simulink model "AppMain"  (R2023a)
settings: Solver=FixedStepDiscrete  StartTime=0.0  StopTime=0.02  FixedStep=10e-3  RelTol=1e-3
PreLoadFcn:
  | AppMain_data
values from neighbouring files (symbols this model uses):
  CtrlConst = struct    [AppMain_data.m]
  TaskTimeBase = struct    [AppMain_data.m]
libraries: simulink x23, lib1 x6
(part 2 of 2)

== system AppMain/FeedBack/Subsystem7/Subsystem5 ==
  FaultFlag : Inport  OutDataTypeStr=boolean
  FaultCnt : Inport  Port=2  OutDataTypeStr=uint8
  MotorRunEn : Inport  Port=3
  Compare To Constant : simulink/Logic and Bit Operations/Compare To Constant  relop=>=  const=2  OutDataTypeStr=boolean
  Logical Operator : Logic  AllPortsSameDT=off  OutDataTypeStr=boolean
  Logical Operator3 : Logic  AllPortsSameDT=off  OutDataTypeStr=boolean
  FeedBackEn : Outport  VectorParamsAs1DForOutWhenUnconnected=off
  wires:
  Compare To Constant/1 -> Logical Operator3/2
  Logical Operator3/1 -> Logical Operator/1
  Logical Operator/1 -> FeedBackEn/1
  MotorRunEn/1 -> Logical Operator/2
  FaultCnt/1 -> Compare To Constant/1
  FaultFlag/1 -> Logical Operator3/1

== system AppMain/FeedBack/Subsystem7/Subsystem6 ==
  FaultFlag : Inport  OutDataTypeStr=boolean
  MotorRunEn : Inport  Port=2
  MDryRunningCnt : Inport  Port=3  OutDataTypeStr=uint8
  Compare To Constant : simulink/Logic and Bit Operations/Compare To Constant  relop=>=  const=2  OutDataTypeStr=boolean
  Logical Operator : Logic  AllPortsSameDT=off  OutDataTypeStr=boolean
  Logical Operator3 : Logic  AllPortsSameDT=off  OutDataTypeStr=boolean
  FeedBackEn : Outport  VectorParamsAs1DForOutWhenUnconnected=off
  wires:
  MotorRunEn/1 -> Logical Operator/2
  Logical Operator/1 -> FeedBackEn/1
  FaultFlag/1 -> Logical Operator3/1
  Logical Operator3/1 -> Logical Operator/1
  Compare To Constant/1 -> Logical Operator3/2
  MDryRunningCnt/1 -> Compare To Constant/1

== system AppMain/MotorRestartAndFaultCnt/MotorFalutHandle/MotorFaultRecoverTimer ==
  RestartInterval : Inport  OutDataTypeStr=uint16
  MotorRestartCompleted : Inport  Port=2
  MotorRestartFSM : Stateflow chart  TreatAsAtomicUnit=on
  RecoverEnable : Outport  VectorParamsAs1DForOutWhenUnconnected=off
  wires:
  MotorRestartCompleted/1 -> MotorRestartFSM/2(MotorRestartCompleted)
  MotorRestartFSM/1(RecoverEn) -> RecoverEnable/1
  RestartInterval/1 -> MotorRestartFSM/1(TimeTHR)

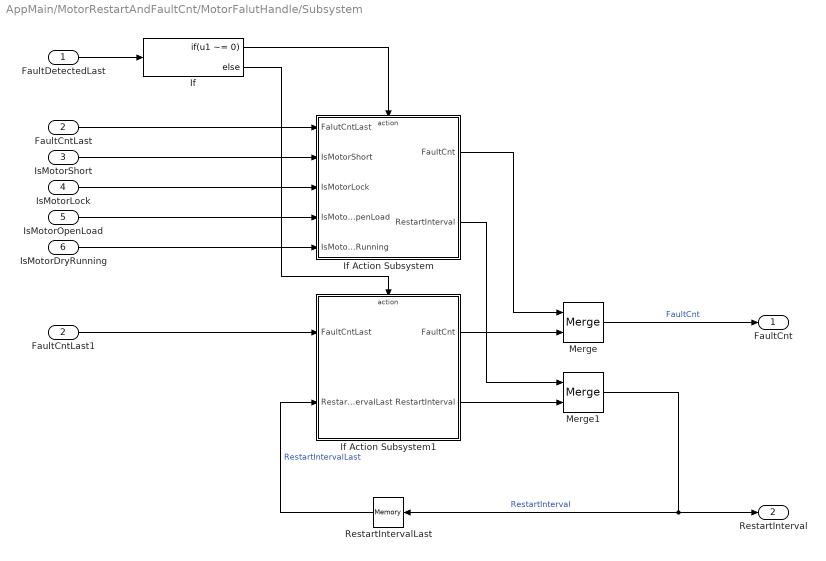
== system AppMain/MotorRestartAndFaultCnt/MotorFalutHandle/Subsystem ==
  FaultDetectedLast : Inport  OutDataTypeStr=boolean
  FaultCntLast : Inport  Port=2  OutDataTypeStr=Bus: MotorFaultCnt_t
  IsMotorShort : Inport  Port=3  OutDataTypeStr=boolean
  IsMotorLock : Inport  Port=4  OutDataTypeStr=boolean
  IsMotorOpenLoad : Inport  Port=5  OutDataTypeStr=boolean
  IsMotorDryRunning : Inport  Port=6  OutDataTypeStr=boolean
  FaultCntLast1 : InportShadow  Port=2  OutDataTypeStr=Bus: MotorFaultCnt_t
  If : If  IfExpression=u1 ~= 0
  If Action Subsystem : Subsystem  TreatAsAtomicUnit=on
  If Action Subsystem1 : Subsystem  TreatAsAtomicUnit=on
  Merge : Merge
  Merge1 : Merge
  RestartIntervalLast : Memory  InheritSampleTime=on
  FaultCnt : Outport  OutDataTypeStr=Bus: MotorFaultCnt_t  VectorParamsAs1DForOutWhenUnconnected=off
  RestartInterval : Outport  Port=2  OutDataTypeStr=uint16  VectorParamsAs1DForOutWhenUnconnected=off
  wires:
  RestartIntervalLast/1 -> If Action Subsystem1/2(RestartIntervalLast)  "RestartIntervalLast"
  If Action Subsystem1/2(RestartInterval) -> Merge1/2
  If Action Subsystem1/1(FaultCnt) -> Merge/2
  If/1 -> If Action Subsystem/Action
  If/2 -> If Action Subsystem1/Action
  Merge1/1 -> RestartIntervalLast/1, RestartInterval/1  "RestartInterval"
  FaultCntLast/1 -> If Action Subsystem/1(FalutCntLast)
  If Action Subsystem/1(FaultCnt) -> Merge/1
  Merge/1 -> FaultCnt/1  "FaultCnt"
  If Action Subsystem/2(RestartInterval) -> Merge1/1
  FaultDetectedLast/1 -> If/1
  IsMotorShort/1 -> If Action Subsystem/2(IsMotorShort)
  IsMotorLock/1 -> If Action Subsystem/3(IsMotorLock)
  IsMotorOpenLoad/1 -> If Action Subsystem/4(IsMotorOpenLoad)
  FaultCntLast1/1 -> If Action Subsystem1/1(FaultCntLast)
  IsMotorDryRunning/1 -> If Action Subsystem/5(IsMotorDryRunning)

== system AppMain/MotorRestartAndFaultCnt/MotorFalutHandle/Subsystem1 ==
  IsMotorShort : Inport  OutDataTypeStr=boolean
  IsMotorOpenLoad : Inport  Port=2  OutDataTypeStr=boolean
  TargetSpeed : Inport  Port=3  OutDataTypeStr=int16
  RestartEnable : Inport  Port=4  OutDataTypeStr=boolean
  IsMotorLock : Inport  Port=5  OutDataTypeStr=boolean
  If : If  NumInputs=2  IfExpression=u1 ~= 0  ElseIfExpressions=u2 ~= 0
  If Action Subsystem : Subsystem  TreatAsAtomicUnit=on
  If Action Subsystem1 : Subsystem  TreatAsAtomicUnit=on
  If Action Subsystem2 : Subsystem  TreatAsAtomicUnit=on
  Logical Operator : Logic  Operator=OR  AllPortsSameDT=off  OutDataTypeStr=boolean
  Merge : Merge  Inputs=3
  Scope : Scope
  Speed : Outport  OutDataTypeStr=int16  VectorParamsAs1DForOutWhenUnconnected=off
  wires:
  IsMotorShort/1 -> Logical Operator/1
  IsMotorOpenLoad/1 -> Logical Operator/2
  Logical Operator/1 -> If/1
  TargetSpeed/1 -> If Action Subsystem2/2(SpeedIn), If Action Subsystem1/1(SpeedIn), If Action Subsystem/1(SpeedIn)
  RestartEnable/1 -> If Action Subsystem2/1(RestartEnable), If Action Subsystem1/2(RestartEnable)
  If/1 -> If Action Subsystem/Action
  If Action Subsystem1/1(SpeedOut) -> Merge/2
  If Action Subsystem/1(SpeedOut) -> Merge/1
  Merge/1 -> Speed/1, Scope/1
  IsMotorLock/1 -> If/2
  If/2 -> If Action Subsystem1/Action
  If/3 -> If Action Subsystem2/Action
  If Action Subsystem2/1(SpeedOut) -> Merge/3

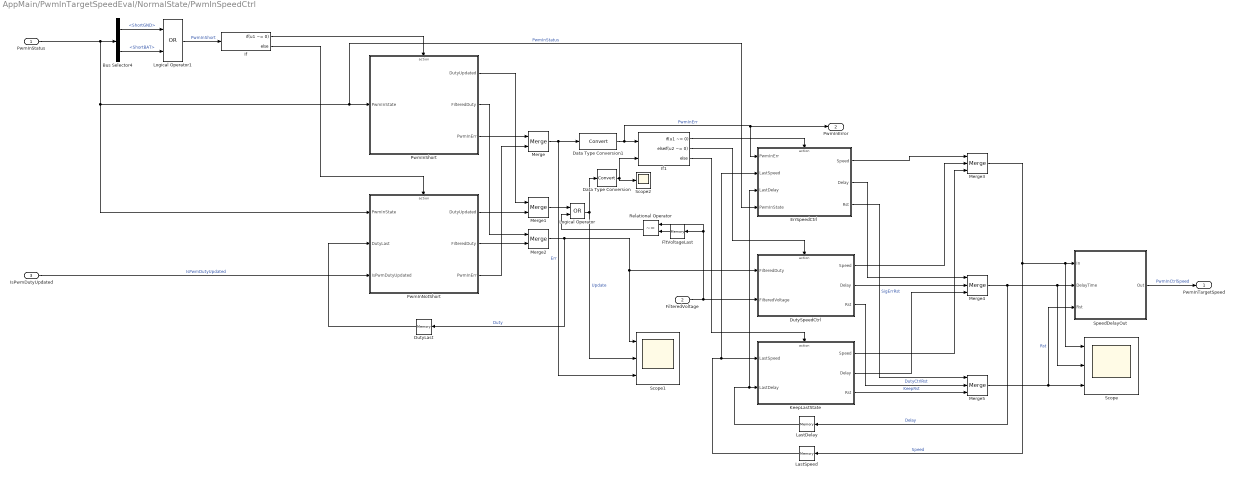
== system AppMain/PwmInTargetSpeedEval/NormalState/PwmInSpeedCtrl ==
  PwmInStatus : Inport
  FilteredVoltage : Inport  Port=2  OutDataTypeStr=int16
  IsPwmDutyUpdated : Inport  Port=3  OutDataTypeStr=boolean
  Bus Selector4 : BusSelector  OutputSignals=ShortGND,ShortBAT
  Data Type Conversion : DataTypeConversion  SaturateOnIntegerOverflow=off  RndMeth=Floor
  Data Type Conversion1 : DataTypeConversion  SaturateOnIntegerOverflow=off  RndMeth=Floor
  DutyLast : Memory  InitialCondition=CtrlConst.SpeedCtrl.PwmIn.Duty.Default  InheritSampleTime=on
  DutySpeedCtrl : Subsystem  TreatAsAtomicUnit=on
  ErrSpeedCtrl : Subsystem  TreatAsAtomicUnit=on
  FltVoltageLast : Memory  InheritSampleTime=on
  If : If  IfExpression=u1 ~= 0
  If1 : If  NumInputs=2  IfExpression=u1 ~= 0  ElseIfExpressions=u2 ~= 0
  KeepLastState : Subsystem  TreatAsAtomicUnit=on
  LastDelay : Memory  InheritSampleTime=on
  LastSpeed : Memory  InheritSampleTime=on
  Logical Operator : Logic  Operator=OR  AllPortsSameDT=off  OutDataTypeStr=boolean
  Logical Operator1 : Logic  Operator=OR  AllPortsSameDT=off  OutDataTypeStr=boolean
  Merge : Merge
  Merge1 : Merge
  Merge2 : Merge
  Merge3 : Merge  Inputs=3
  Merge4 : Merge  Inputs=3
  Merge5 : Merge  Inputs=3
  PwmInNotShort : Subsystem  TreatAsAtomicUnit=on
      settings: RTWSystemCode=Nonreusable function  RTWFcnNameOpts=Use subsystem name  FunctionInterfaceSpec=Allow arguments (Optimized)
  PwmInShort : Subsystem  TreatAsAtomicUnit=on
      settings: RTWSystemCode=Nonreusable function  RTWFcnNameOpts=Use subsystem name  FunctionInterfaceSpec=Allow arguments (Optimized)
  Relational Operator : RelationalOperator  Operator=~=  OutDataTypeStr=boolean  RndMeth=Simplest  InputSameDT=off
  Scope : Scope  NumInputPorts=3
  Scope1 : Scope  NumInputPorts=3
  Scope2 : Scope
  SpeedDelayOut : Subsystem  TreatAsAtomicUnit=on
      settings: RTWFcnNameOpts=Use subsystem name
  PwmInTargetSpeed : Outport  VectorParamsAs1DForOutWhenUnconnected=off
  PwmInError : Outport  Port=2  OutDataTypeStr=boolean  VectorParamsAs1DForOutWhenUnconnected=off
  wires:
  SpeedDelayOut/1(Out) -> PwmInTargetSpeed/1  "PwmInCtrlSpeed"
  PwmInStatus/1 -> PwmInNotShort/1(PwmInState), ErrSpeedCtrl/4(PwmInState), PwmInShort/1(PwmInState), Bus Selector4/1  "PwmInStatus"
  Bus Selector4/1 -> Logical Operator1/1  "<ShortGND>"
  Bus Selector4/2 -> Logical Operator1/2  "<ShortBAT>"
  Logical Operator1/1 -> If/1  "PwmInShort"
  If/1 -> PwmInShort/Action
  If/2 -> PwmInNotShort/Action
  PwmInShort/3(PwmInErr) -> Merge/1
  PwmInNotShort/3(PwmInErr) -> Merge/2
  If1/1 -> ErrSpeedCtrl/Action
  PwmInNotShort/1(DutyUpdated) -> Merge1/2
  PwmInShort/1(DutyUpdated) -> Merge1/1
  PwmInNotShort/2(FilteredDuty) -> Merge2/2
  PwmInShort/2(FilteredDuty) -> Merge2/1
  Merge2/1 -> DutyLast/1, Scope1/1, DutySpeedCtrl/1(FilteredDuty)  "Duty"
  ErrSpeedCtrl/1(Speed) -> Merge3/1
  DutySpeedCtrl/1(Speed) -> Merge3/2
  ErrSpeedCtrl/2(Delay) -> Merge4/1
  DutySpeedCtrl/2(Delay) -> Merge4/2
  ErrSpeedCtrl/3(Rst) -> Merge5/1  "SigErrRst"
  DutySpeedCtrl/3(Rst) -> Merge5/2  "DutyCtrlRst"
  Merge3/1 -> SpeedDelayOut/1(In), Scope/1, LastSpeed/1  "Speed"
  Merge4/1 -> Scope/2, SpeedDelayOut/2(DelayTime), LastDelay/1  "Delay"
  Merge5/1 -> Scope/3, SpeedDelayOut/3(Rst)  "Rst"
  If1/2 -> DutySpeedCtrl/Action
  Merge1/1 -> Logical Operator/1
  If1/3 -> KeepLastState/Action
  LastDelay/1 -> ErrSpeedCtrl/3(LastDelay), KeepLastState/2(LastDelay)
  LastSpeed/1 -> ErrSpeedCtrl/2(LastSpeed), KeepLastState/1(LastSpeed)
  KeepLastState/3(Rst) -> Merge5/3  "KeepRst"
  KeepLastState/2(Delay) -> Merge4/3
  KeepLastState/1(Speed) -> Merge3/3
  Data Type Conversion1/1 -> ErrSpeedCtrl/1(PwmInErr), PwmInError/1, If1/1  "PwmInErr"
  Data Type Conversion/1 -> If1/2, Scope2/1
  DutyLast/1 -> PwmInNotShort/2(DutyLast)
  FltVoltageLast/1 -> Relational Operator/2
  FilteredVoltage/1 -> FltVoltageLast/1, Relational Operator/1, DutySpeedCtrl/2(FilteredVoltage)
  Relational Operator/1 -> Logical Operator/2
  Merge/1 -> Data Type Conversion1/1, Scope1/3  "Err"
  Logical Operator/1 -> Scope1/2, Data Type Conversion/1  "Update"
  IsPwmDutyUpdated/1 -> PwmInNotShort/3(IsPwmDutyUpdated)  "IsPwmDutyUpdated"

== system AppMain/MotorRestartAndFaultCnt/MotorFalutHandle/Subsystem/If Action Subsystem ==
  FalutCntLast : Inport  OutDataTypeStr=Bus: MotorFaultCnt_t
  IsMotorShort : Inport  Port=2  OutDataTypeStr=boolean
  IsMotorLock : Inport  Port=3  OutDataTypeStr=boolean
  IsMotorOpenLoad : Inport  Port=4  OutDataTypeStr=boolean
  IsMotorDryRunning : Inport  Port=5  OutDataTypeStr=boolean
  Action Port : ActionPort  InitializeStates=reset  ActionPortLabel=if(u1 ~= 0)
  FaultCntIncrement : Subsystem
  RestartIntervalCaculate : Subsystem
  FaultCnt : Outport  OutDataTypeStr=Bus: MotorFaultCnt_t  VectorParamsAs1DForOutWhenUnconnected=off
  RestartInterval : Outport  Port=2  OutDataTypeStr=uint16  VectorParamsAs1DForOutWhenUnconnected=off
  wires:
  FaultCntIncrement/1(FaultCnt) -> RestartIntervalCaculate/1(MotorFaultCnt), FaultCnt/1
  FalutCntLast/1 -> FaultCntIncrement/1(FalutCntLast)
  IsMotorShort/1 -> FaultCntIncrement/2(IsMotorShort)
  RestartIntervalCaculate/1(TimeTHR) -> RestartInterval/1
  IsMotorOpenLoad/1 -> FaultCntIncrement/3(IsMotorOpenLoad)
  IsMotorLock/1 -> FaultCntIncrement/4(IsMotorLock)
  IsMotorDryRunning/1 -> FaultCntIncrement/5(IsMotorDryRunning)

== system AppMain/MotorRestartAndFaultCnt/MotorFalutHandle/Subsystem/If Action Subsystem1 ==
  FaultCntLast : Inport  OutDataTypeStr=Bus: MotorFaultCnt_t
  RestartIntervalLast : Inport  Port=2  OutDataTypeStr=uint16
  Action Port : ActionPort  InitializeStates=reset  ActionPortLabel=else
  Bus Creator : BusCreator  Inputs=4  OutDataTypeStr=Bus: MotorFaultCnt_t  NonVirtualBus=on
      settings: InheritFromInputs=off
  Bus Selector : BusSelector  OutputSignals=Short,Open,Lock,DryRunning
  FaultCnt : Outport  OutDataTypeStr=Bus: MotorFaultCnt_t  VectorParamsAs1DForOutWhenUnconnected=off
  RestartInterval : Outport  Port=2  OutDataTypeStr=uint16  VectorParamsAs1DForOutWhenUnconnected=off
  wires:
  FaultCntLast/1 -> Bus Selector/1
  Bus Creator/1 -> FaultCnt/1
  Bus Selector/1 -> Bus Creator/1  "<Short>"
  Bus Selector/2 -> Bus Creator/2  "<Open>"
  Bus Selector/3 -> Bus Creator/3  "<Lock>"
  RestartIntervalLast/1 -> RestartInterval/1
  Bus Selector/4 -> Bus Creator/4  "<DryRunning>"

== system AppMain/MotorRestartAndFaultCnt/MotorFalutHandle/Subsystem1/If Action Subsystem ==
  SpeedIn : Inport
  Action Port : ActionPort  ActionPortLabel=if(u1 ~= 0)
  SpeedOut : Outport  VectorParamsAs1DForOutWhenUnconnected=off
  wires:
  SpeedIn/1 -> SpeedOut/1

== system AppMain/MotorRestartAndFaultCnt/MotorFalutHandle/Subsystem1/If Action Subsystem1 ==
  SpeedIn : Inport
  RestartEnable : Inport  Port=2  OutDataTypeStr=boolean
  Action Port : ActionPort  InitializeStates=reset  ActionPortLabel=elseif(u2 ~= 0)
  Add : Sum  SaturateOnIntegerOverflow=on
  Compare To Constant : simulink/Logic and Bit Operations/Compare To Constant  relop=<=  const=2/5e-3  OutDataTypeStr=boolean
  Constant : Constant  Value=0  OutDataTypeStr=uint16
  Constant1 : Constant  OutDataTypeStr=uint16
  Constant2 : Constant  Value=-1000  OutDataTypeStr=int16
  Detect Increase : simulink/Logic and Bit Operations/Detect Increase  vinit=0.0  OutDataTypeStr=boolean
  Memory : Memory  InitialCondition=uint16(0)  InheritSampleTime=on
  Scope : Scope  NumInputPorts=2
  Switch : Switch  Criteria=u2 > Threshold  SaturateOnIntegerOverflow=off  InputSameDT=off
  Switch1 : Switch  Criteria=u2 > Threshold  SaturateOnIntegerOverflow=off  InputSameDT=off
  SpeedOut : Outport  VectorParamsAs1DForOutWhenUnconnected=off
  wires:
  RestartEnable/1 -> Detect Increase/1
  Detect Increase/1 -> Switch/2
  Switch/1 -> Memory/1, Compare To Constant/1
  Memory/1 -> Add/2
  Constant/1 -> Switch/1
  Add/1 -> Switch/3
  Constant1/1 -> Add/1
  Compare To Constant/1 -> Switch1/2, Scope/2
  Constant2/1 -> Switch1/1
  Switch1/1 -> SpeedOut/1, Scope/1
  SpeedIn/1 -> Switch1/3

== system AppMain/MotorRestartAndFaultCnt/MotorFalutHandle/Subsystem1/If Action Subsystem2 ==
  RestartEnable : Inport  OutDataTypeStr=boolean
  SpeedIn : Inport  Port=2
  Action Port : ActionPort  InitializeStates=reset  ActionPortLabel=else
  Constant : Constant  Value=0  OutDataTypeStr=int16
  Switch : Switch  Criteria=u2 > Threshold  SaturateOnIntegerOverflow=off  InputSameDT=off
  SpeedOut : Outport  VectorParamsAs1DForOutWhenUnconnected=off
  wires:
  Switch/1 -> SpeedOut/1
  Constant/1 -> Switch/3
  RestartEnable/1 -> Switch/2
  SpeedIn/1 -> Switch/1

== system AppMain/PwmInTargetSpeedEval/NormalState/PwmInSpeedCtrl/DutySpeedCtrl ==
  FilteredDuty : Inport  OutDataTypeStr=uint16
  FilteredVoltage : Inport  Port=2  OutDataTypeStr=int16
  Action Port : ActionPort  InitializeStates=reset  ActionPortLabel=elseif(u2 ~= 0)
  Scope : Scope
  SpeedAndOutDelayEval : Subsystem
      settings: RTWFcnNameOpts=Use subsystem name
  Speed : Outport  OutDataTypeStr=int16  VectorParamsAs1DForOutWhenUnconnected=off
  Delay : Outport  Port=2  OutDataTypeStr=uint16  VectorParamsAs1DForOutWhenUnconnected=off
  Rst : Outport  Port=3  OutDataTypeStr=boolean  VectorParamsAs1DForOutWhenUnconnected=off
  wires:
  FilteredDuty/1 -> SpeedAndOutDelayEval/1(FilteredDuty)
  SpeedAndOutDelayEval/1(DutySpeed) -> Speed/1  "Speed"
  SpeedAndOutDelayEval/2(DelayTime) -> Delay/1  "Delay"
  SpeedAndOutDelayEval/3(DelayRst) -> Rst/1, Scope/1  "Rst"
  FilteredVoltage/1 -> SpeedAndOutDelayEval/2(FilteredVoltage)

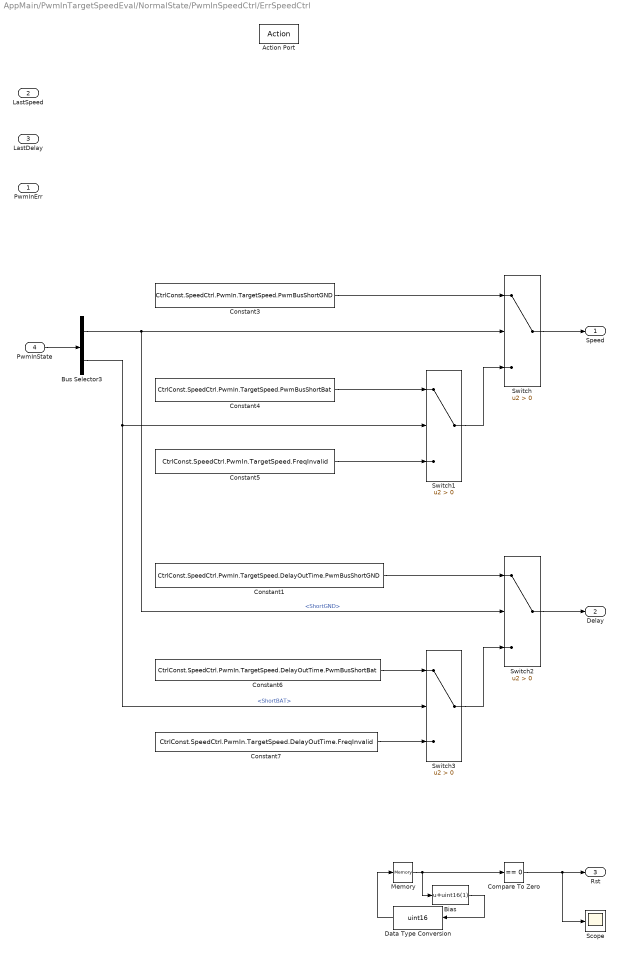
== system AppMain/PwmInTargetSpeedEval/NormalState/PwmInSpeedCtrl/ErrSpeedCtrl ==
  PwmInErr : Inport  OutDataTypeStr=boolean
  LastSpeed : Inport  Port=2  OutDataTypeStr=int16
  LastDelay : Inport  Port=3  OutDataTypeStr=uint16
  PwmInState : Inport  Port=4
  Action Port : ActionPort  InitializeStates=reset  ActionPortLabel=if(u1 ~= 0)
  Bias : Bias  Bias=uint16(1)  SaturateOnIntegerOverflow=off
  Bus Selector3 : BusSelector  OutputSignals=ShortGND,ShortBAT
  Compare To Zero : simulink/Logic and Bit Operations/Compare To Zero  relop===  OutDataTypeStr=boolean
  Constant1 : Constant  Value=CtrlConst.SpeedCtrl.PwmIn.TargetSpeed.DelayOutTime.PwmBusShortGND
  Constant3 : Constant  Value=CtrlConst.SpeedCtrl.PwmIn.TargetSpeed.PwmBusShortGND
  Constant4 : Constant  Value=CtrlConst.SpeedCtrl.PwmIn.TargetSpeed.PwmBusShortBat
  Constant5 : Constant  Value=CtrlConst.SpeedCtrl.PwmIn.TargetSpeed.FreqInvalid
  Constant6 : Constant  Value=CtrlConst.SpeedCtrl.PwmIn.TargetSpeed.DelayOutTime.PwmBusShortBat
  Constant7 : Constant  Value=CtrlConst.SpeedCtrl.PwmIn.TargetSpeed.DelayOutTime.FreqInvalid
  Data Type Conversion : DataTypeConversion  OutDataTypeStr=uint16  SaturateOnIntegerOverflow=off  RndMeth=Floor
  Memory : Memory  InitialCondition=uint16(0)  InheritSampleTime=on
  Scope : Scope
  Switch{,1..3} (4 alike) : Switch  Criteria=u2 > Threshold  SaturateOnIntegerOverflow=off  InputSameDT=off
  Speed : Outport  OutDataTypeStr=int16  VectorParamsAs1DForOutWhenUnconnected=off
  Delay : Outport  Port=2  OutDataTypeStr=uint16  VectorParamsAs1DForOutWhenUnconnected=off
  Rst : Outport  Port=3  OutDataTypeStr=boolean  VectorParamsAs1DForOutWhenUnconnected=off
  wires:
  PwmInState/1 -> Bus Selector3/1
  Constant3/1 -> Switch/1
  Switch1/1 -> Switch/3
  Constant4/1 -> Switch1/1
  Constant5/1 -> Switch1/3
  Switch/1 -> Speed/1
  Switch3/1 -> Switch2/3
  Bus Selector3/2 -> Switch3/2, Switch1/2  "<ShortBAT>"
  Constant1/1 -> Switch2/1
  Bus Selector3/1 -> Switch2/2, Switch/2  "<ShortGND>"
  Constant7/1 -> Switch3/3
  Constant6/1 -> Switch3/1
  Switch2/1 -> Delay/1
  Data Type Conversion/1 -> Memory/1
  Bias/1 -> Data Type Conversion/1
  Memory/1 -> Bias/1, Compare To Zero/1
  Compare To Zero/1 -> Rst/1, Scope/1

== system AppMain/PwmInTargetSpeedEval/NormalState/PwmInSpeedCtrl/KeepLastState ==
  LastSpeed : Inport  OutDataTypeStr=int16
  LastDelay : Inport  Port=2  OutDataTypeStr=uint16
  Action Port : ActionPort  InitializeStates=reset  ActionPortLabel=else
  Constant : Constant  Value=false  OutDataTypeStr=boolean
  Speed : Outport  OutDataTypeStr=int16  VectorParamsAs1DForOutWhenUnconnected=off
  Delay : Outport  Port=2  OutDataTypeStr=uint16  VectorParamsAs1DForOutWhenUnconnected=off
  Rst : Outport  Port=3  OutDataTypeStr=boolean  VectorParamsAs1DForOutWhenUnconnected=off
  wires:
  LastSpeed/1 -> Speed/1
  LastDelay/1 -> Delay/1
  Constant/1 -> Rst/1

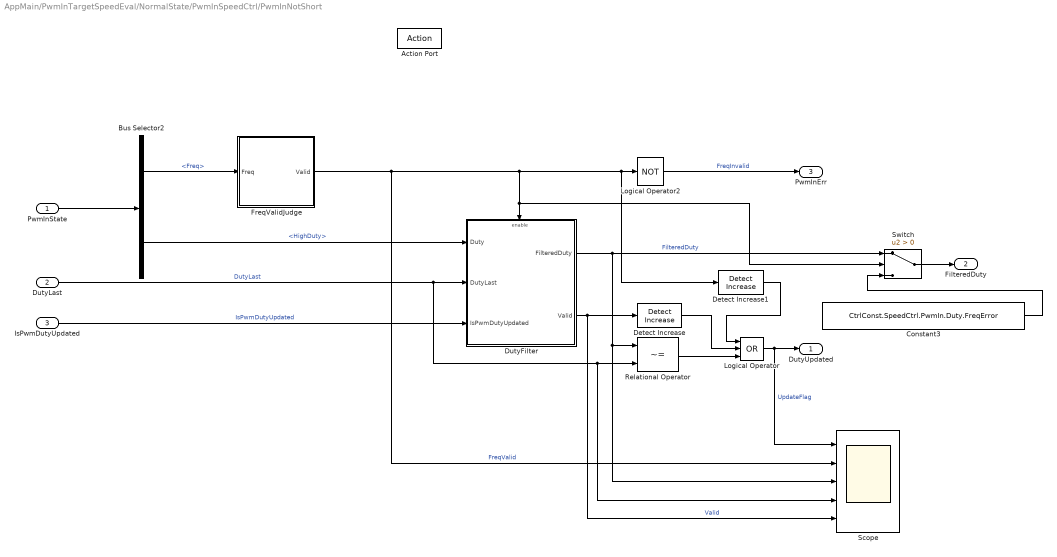
== system AppMain/PwmInTargetSpeedEval/NormalState/PwmInSpeedCtrl/PwmInNotShort ==
  PwmInState : Inport
  DutyLast : Inport  Port=2  OutDataTypeStr=uint16
  IsPwmDutyUpdated : Inport  Port=3  OutDataTypeStr=boolean
  Action Port : ActionPort  InitializeStates=reset  ActionPortLabel=else
  Bus Selector2 : BusSelector  OutputSignals=Freq,HighDuty
  Constant3 : Constant  Value=CtrlConst.SpeedCtrl.PwmIn.Duty.FreqError
  Detect Increase : simulink/Logic and Bit Operations/Detect Increase  vinit=0.0  OutDataTypeStr=boolean
  Detect Increase1 : simulink/Logic and Bit Operations/Detect Increase  vinit=0.0  OutDataTypeStr=boolean
  DutyFilter : Subsystem  TreatAsAtomicUnit=on
      settings: RTWFcnNameOpts=Use subsystem name
  FreqValidJudge : Subsystem  TreatAsAtomicUnit=on
      settings: RTWFcnNameOpts=Use subsystem name
  Logical Operator : Logic  Operator=OR  Inputs=3  AllPortsSameDT=off  OutDataTypeStr=boolean
  Logical Operator2 : Logic  Operator=NOT  Inputs=3  AllPortsSameDT=off  OutDataTypeStr=boolean
  Relational Operator : RelationalOperator  Operator=~=  OutDataTypeStr=boolean  RndMeth=Simplest  InputSameDT=off
  Scope : Scope  NumInputPorts=5
  Switch : Switch  Criteria=u2 > Threshold  SaturateOnIntegerOverflow=off  InputSameDT=off
  DutyUpdated : Outport  OutDataTypeStr=boolean  VectorParamsAs1DForOutWhenUnconnected=off
  FilteredDuty : Outport  Port=2  OutDataTypeStr=uint16  VectorParamsAs1DForOutWhenUnconnected=off
  PwmInErr : Outport  Port=3  OutDataTypeStr=boolean  VectorParamsAs1DForOutWhenUnconnected=off
  wires:
  Detect Increase/1 -> Logical Operator/2
  DutyFilter/2(Valid) -> Scope/5, Detect Increase/1  "Valid"
  PwmInState/1 -> Bus Selector2/1
  Bus Selector2/2 -> DutyFilter/1(Duty)  "<HighDuty>"
  Bus Selector2/1 -> FreqValidJudge/1(Freq)  "<Freq>"
  DutyFilter/1(FilteredDuty) -> Switch/1, Relational Operator/1, Scope/3  "FilteredDuty"
  Logical Operator2/1 -> PwmInErr/1  "FreqInvalid"
  FreqValidJudge/1(Valid) -> Detect Increase1/1, Logical Operator2/1, Switch/2, DutyFilter/Enable, Scope/2  "FreqValid"
  DutyLast/1 -> Relational Operator/2, Scope/4, DutyFilter/2(DutyLast)  "DutyLast"
  Relational Operator/1 -> Logical Operator/3
  Logical Operator/1 -> DutyUpdated/1, Scope/1  "UpdateFlag"
  IsPwmDutyUpdated/1 -> DutyFilter/3(IsPwmDutyUpdated)  "IsPwmDutyUpdated"
  Detect Increase1/1 -> Logical Operator/1
  Switch/1 -> FilteredDuty/1
  Constant3/1 -> Switch/3

== system AppMain/PwmInTargetSpeedEval/NormalState/PwmInSpeedCtrl/PwmInShort ==
  PwmInState : Inport
  Action Port : ActionPort  InitializeStates=reset  ActionPortLabel=if(u1 ~= 0)
  Bus Selector3 : BusSelector  OutputSignals=ShortGND,ShortBAT
  Constant : Constant  OutDataTypeStr=boolean
  Detect Increase : simulink/Logic and Bit Operations/Detect Increase  vinit=0.0  OutDataTypeStr=boolean
  Detect Increase1 : simulink/Logic and Bit Operations/Detect Increase  vinit=0.0  OutDataTypeStr=boolean
  Duty0 : Constant  Value=0  OutDataTypeStr=uint16
  Duty100 : Constant  Value=1000  OutDataTypeStr=uint16
  Logical Operator3 : Logic  Operator=OR  AllPortsSameDT=off  OutDataTypeStr=boolean
  Switch : Switch  Criteria=u2 > Threshold  SaturateOnIntegerOverflow=off  InputSameDT=off
  DutyUpdated : Outport  OutDataTypeStr=boolean  VectorParamsAs1DForOutWhenUnconnected=off
  FilteredDuty : Outport  Port=2  OutDataTypeStr=uint16  VectorParamsAs1DForOutWhenUnconnected=off
  PwmInErr : Outport  Port=3  OutDataTypeStr=boolean  VectorParamsAs1DForOutWhenUnconnected=off
  wires:
  Switch/1 -> FilteredDuty/1  "FilteredDuty"
  Logical Operator3/1 -> DutyUpdated/1  "DutyUpdate"
  Bus Selector3/2 -> Detect Increase1/1, Switch/2  "<ShortBAT>"
  Bus Selector3/1 -> Detect Increase/1  "<ShortGND>"
  Detect Increase1/1 -> Logical Operator3/2
  Detect Increase/1 -> Logical Operator3/1
  Duty0/1 -> Switch/3
  Duty100/1 -> Switch/1
  PwmInState/1 -> Bus Selector3/1
  Constant/1 -> PwmInErr/1

== system AppMain/PwmInTargetSpeedEval/NormalState/PwmInSpeedCtrl/SpeedDelayOut ==
  In : Inport
  DelayTime : Inport  Port=2
  Rst : Inport  Port=3
  DelayOut : Stateflow chart  TreatAsAtomicUnit=on
  OutLast : Memory  InheritSampleTime=on
  Out : Outport  VectorParamsAs1DForOutWhenUnconnected=off
  wires:
  In/1 -> DelayOut/1(In)  "In"
  OutLast/1 -> DelayOut/4(OutLast)  "OutLast"
  Rst/1 -> DelayOut/3(Rst)  "Rst"
  DelayOut/1(Out) -> OutLast/1, Out/1  "Out"
  DelayTime/1 -> DelayOut/2(DelayTHR)  "DelayTHR"

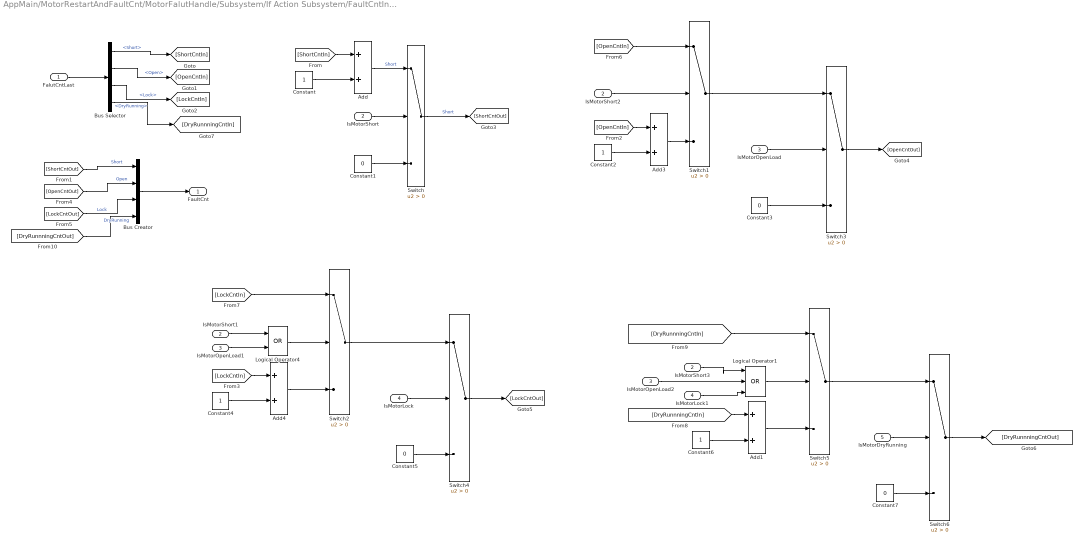
== system AppMain/MotorRestartAndFaultCnt/MotorFalutHandle/Subsystem/If Action Subsystem/FaultCntIncrement ==
  FalutCntLast : Inport  OutDataTypeStr=Bus: MotorFaultCnt_t
  IsMotorShort : Inport  Port=2  OutDataTypeStr=boolean
  IsMotorOpenLoad : Inport  Port=3  OutDataTypeStr=boolean
  IsMotorLock : Inport  Port=4  OutDataTypeStr=boolean
  IsMotorDryRunning : Inport  Port=5  OutDataTypeStr=boolean
  Add{,1,3..4} (4 alike) : Sum  SaturateOnIntegerOverflow=on
  Bus Creator : BusCreator  Inputs=4  OutDataTypeStr=Bus: MotorFaultCnt_t  NonVirtualBus=on
      settings: InheritFromInputs=off
  Bus Selector : BusSelector  OutputSignals=Short,Open,Lock,DryRunning
  Constant{,2,4,6} (4 alike) : Constant  OutDataTypeStr=uint8
  Constant{1,3,5,7} (4 alike) : Constant  Value=0  OutDataTypeStr=uint8
  IsMotorLock1 : InportShadow  Port=4  OutDataTypeStr=boolean
  IsMotorOpenLoad1 : InportShadow  Port=3  OutDataTypeStr=boolean
  IsMotorOpenLoad2 : InportShadow  Port=3  OutDataTypeStr=boolean
  IsMotorShort1 : InportShadow  Port=2  OutDataTypeStr=boolean
  IsMotorShort2 : InportShadow  Port=2  OutDataTypeStr=boolean
  IsMotorShort3 : InportShadow  Port=2  OutDataTypeStr=boolean
  Logical Operator1 : Logic  Operator=OR  Inputs=3  AllPortsSameDT=off  OutDataTypeStr=boolean
  Logical Operator4 : Logic  Operator=OR  AllPortsSameDT=off  OutDataTypeStr=boolean
  Switch{,1..6} (7 alike) : Switch  Criteria=u2 > Threshold  SaturateOnIntegerOverflow=off  InputSameDT=off
  FaultCnt : Outport  OutDataTypeStr=Bus: MotorFaultCnt_t  VectorParamsAs1DForOutWhenUnconnected=off
  wires:
  Bus Creator/1 -> FaultCnt/1
  Constant/1 -> Add/2
  Bus Selector/2 -> [OpenCntIn]  "<Open>"
  Bus Selector/1 -> [ShortCntIn]  "<Short>"
  Constant1/1 -> Switch/3
  Add/1 -> Switch/1  "Short"
  FalutCntLast/1 -> Bus Selector/1
  IsMotorShort/1 -> Switch/2
  Bus Selector/3 -> [LockCntIn]  "<Lock>"
  [ShortCntIn] -> Add/1
  Switch/1 -> [ShortCntOut]  "Short"
  [ShortCntOut] -> Bus Creator/1  "Short"
  Add3/1 -> Switch1/3
  Constant2/1 -> Add3/2
  [OpenCntIn] -> Add3/1
  Constant3/1 -> Switch3/3
  Switch3/1 -> [OpenCntOut]
  IsMotorShort1/1 -> Logical Operator4/1
  Switch4/1 -> [LockCntOut]
  [LockCntIn] -> Add4/1
  Constant4/1 -> Add4/2
  Constant5/1 -> Switch4/3
  IsMotorOpenLoad1/1 -> Logical Operator4/2
  [OpenCntOut] -> Bus Creator/2  "Open"
  [LockCntOut] -> Bus Creator/3  "Lock"
  IsMotorOpenLoad/1 -> Switch3/2
  IsMotorShort2/1 -> Switch1/2
  [OpenCntIn] -> Switch1/1
  Switch1/1 -> Switch3/1
  IsMotorLock/1 -> Switch4/2
  Switch2/1 -> Switch4/1
  Logical Operator4/1 -> Switch2/2
  [LockCntIn] -> Switch2/1
  Add4/1 -> Switch2/3
  Add1/1 -> Switch5/3
  Logical Operator1/1 -> Switch5/2
  [DryRunnningCntIn] -> Switch5/1
  [DryRunnningCntIn] -> Add1/1
  IsMotorDryRunning/1 -> Switch6/2
  Constant7/1 -> Switch6/3
  Switch5/1 -> Switch6/1
  Constant6/1 -> Add1/2
  Switch6/1 -> [DryRunnningCntOut]
  IsMotorShort3/1 -> Logical Operator1/1
  IsMotorLock1/1 -> Logical Operator1/3
  IsMotorOpenLoad2/1 -> Logical Operator1/2
  Bus Selector/4 -> [DryRunnningCntIn]  "<DryRunning>"
  [DryRunnningCntOut] -> Bus Creator/4  "DryRunning"

== system AppMain/MotorRestartAndFaultCnt/MotorFalutHandle/Subsystem/If Action Subsystem/RestartIntervalCaculate ==
  MotorFaultCnt : Inport  OutDataTypeStr=Bus: MotorFaultCnt_t
  Bus Selector : BusSelector  OutputSignals=Short,Open,Lock,DryRunning
  Dryrunning : Subsystem  TreatAsAtomicUnit=on
  If : If  NumInputs=3  ElseIfExpressions=u2 > 0,u3 > 0
  Lock : Subsystem  TreatAsAtomicUnit=on
  Merge : Merge  Inputs=4
  Open : Subsystem  TreatAsAtomicUnit=on
  Scope : Scope  NumInputPorts=4
  Short : Subsystem  TreatAsAtomicUnit=on
  TimeTHR : Outport  OutDataTypeStr=uint16  VectorParamsAs1DForOutWhenUnconnected=off
  wires:
  Bus Selector/1 -> If/1, Scope/2, Short/1(FaultCnt)  "<Short>"
  Bus Selector/3 -> Lock/1(FaultCnt), Scope/4, If/3  "<Lock>"
  Bus Selector/2 -> Open/1(FaultCnt), Scope/3, If/2  "<Open>"
  MotorFaultCnt/1 -> Bus Selector/1
  If/1 -> Short/Action
  If/2 -> Open/Action
  Merge/1 -> TimeTHR/1, Scope/1
  Open/1(Interval) -> Merge/2
  Lock/1(Interval) -> Merge/3
  Short/1(Interval) -> Merge/1
  If/3 -> Lock/Action
  If/4 -> Dryrunning/Action
  Bus Selector/4 -> Dryrunning/1(FaultCnt)  "<DryRunning>"
  Dryrunning/1(Interval) -> Merge/4

== system AppMain/PwmInTargetSpeedEval/NormalState/PwmInSpeedCtrl/DutySpeedCtrl/SpeedAndOutDelayEval ==
  FilteredDuty : Inport
  FilteredVoltage : Inport  Port=2  OutDataTypeStr=int16
  Constant : Constant  Value=CtrlConst.SpeedCtrl.PwmIn.TargetSpeed.Min  OutDataTypeStr=int16
  Data Type Conversion : DataTypeConversion  OutDataTypeStr=uint16  SaturateOnIntegerOverflow=off  RndMeth=Floor
  LastState : Memory  InitialCondition=uint16(0)  InheritSampleTime=on
  MaxSpeedLimtedByVoltage : Subsystem  TreatAsAtomicUnit=on
  SpeedCurve : MATLAB Function  TreatAsAtomicUnit=on
      settings: RTWFcnNameOpts=Use subsystem name
  DutySpeed : Outport  VectorParamsAs1DForOutWhenUnconnected=off
  DelayTime : Outport  Port=2  VectorParamsAs1DForOutWhenUnconnected=off
  DelayRst : Outport  Port=3  OutDataTypeStr=boolean  VectorParamsAs1DForOutWhenUnconnected=off
  wires:
  FilteredDuty/1 -> SpeedCurve/3(Duty)  "FilteredDuty"
  LastState/1 -> Data Type Conversion/1
  SpeedCurve/4(SectorNew) -> LastState/1
  SpeedCurve/1(Speed) -> DutySpeed/1
  SpeedCurve/2(Delay) -> DelayTime/1
  SpeedCurve/3(Reset) -> DelayRst/1
  Data Type Conversion/1 -> SpeedCurve/4(SectorLast)
  MaxSpeedLimtedByVoltage/1(MaxSpeed) -> SpeedCurve/1(MaxSpeed)
  FilteredVoltage/1 -> MaxSpeedLimtedByVoltage/1(Voltage)
  Constant/1 -> SpeedCurve/2(MinSpeed)

== system AppMain/PwmInTargetSpeedEval/NormalState/PwmInSpeedCtrl/PwmInNotShort/DutyFilter ==
  Duty : Inport
  DutyLast : Inport  Port=2  OutDataTypeStr=uint16
  IsPwmDutyUpdated : Inport  Port=3  OutDataTypeStr=boolean
  Enable : EnablePort  StatesWhenEnabling=reset
  DutyBuf : Memory  InitialCondition=uint16(ones(1,6)*2000)  InheritSampleTime=on
  Enabled Subsystem : Subsystem  TreatAsAtomicUnit=on
  Switch : Switch  Criteria=u2 > Threshold  SaturateOnIntegerOverflow=off  InputSameDT=off
  FilteredDuty : Outport  VectorParamsAs1DForOutWhenUnconnected=off
  Valid : Outport  Port=2  VectorParamsAs1DForOutWhenUnconnected=off
  wires:
  Enabled Subsystem/2(Valid) -> Valid/1
  Duty/1 -> Enabled Subsystem/1(Duty)  "Duty"
  DutyLast/1 -> Switch/3, Enabled Subsystem/2(DutyLast)  "DutyLast"
  Enabled Subsystem/1(FilteredDuty) -> Switch/1
  IsPwmDutyUpdated/1 -> Enabled Subsystem/Enable, Switch/2  "IsPwmDutyUpdated"
  Enabled Subsystem/3(DutyBufOut) -> DutyBuf/1
  DutyBuf/1 -> Enabled Subsystem/3(DutyBufIn)
  Switch/1 -> FilteredDuty/1

== system AppMain/PwmInTargetSpeedEval/NormalState/PwmInSpeedCtrl/PwmInNotShort/FreqValidJudge ==
  Freq : Inport
  FreqMax : Constant  Value=CtrlConst.SpeedCtrl.PwmIn.Freq.Max
  FreqMin : Constant  Value=CtrlConst.SpeedCtrl.PwmIn.Freq.Min
  FreqTolerance : Constant  Value=CtrlConst.SpeedCtrl.PwmIn.Freq.Tolerance
  FreqValidJudge : Stateflow chart  TreatAsAtomicUnit=on
  FreqValidJudgeFilterTime : Constant  Value=CtrlConst.SpeedCtrl.PwmIn.Freq.ValidJudgeFilterTime
  Valid : Outport  VectorParamsAs1DForOutWhenUnconnected=off
  wires:
  FreqValidJudge/1(Valid) -> Valid/1
  Freq/1 -> FreqValidJudge/1(Freq)
  FreqMin/1 -> FreqValidJudge/2(FreqMin)
  FreqMax/1 -> FreqValidJudge/3(FreqMax)
  FreqTolerance/1 -> FreqValidJudge/4(FreqTolerance)
  FreqValidJudgeFilterTime/1 -> FreqValidJudge/5(FreqValidJudgeFilterTime)

== system AppMain/MotorRestartAndFaultCnt/MotorFalutHandle/Subsystem/If Action Subsystem/RestartIntervalCaculate/Dryrunning ==
  FaultCnt : Inport
  Action Port : ActionPort  InitializeStates=reset  ActionPortLabel=else
  Constant : Constant  Value=20  OutDataTypeStr=uint16
  Constant1 : Constant  Value=2/TaskTimeBase.SpeedCtrl  OutDataTypeStr=uint16
  Constant2 : Constant  Value=65535  OutDataTypeStr=uint16
  Relational Operator : RelationalOperator  Operator=<  OutDataTypeStr=boolean  RndMeth=Simplest  InputSameDT=off
  Switch5 : Switch  Criteria=u2 > Threshold  SaturateOnIntegerOverflow=off  InputSameDT=off
  Interval : Outport  VectorParamsAs1DForOutWhenUnconnected=off
  wires:
  Constant/1 -> Relational Operator/2
  Relational Operator/1 -> Switch5/2
  Constant2/1 -> Switch5/3
  Constant1/1 -> Switch5/1
  FaultCnt/1 -> Relational Operator/1
  Switch5/1 -> Interval/1  "FaultType"

== system AppMain/MotorRestartAndFaultCnt/MotorFalutHandle/Subsystem/If Action Subsystem/RestartIntervalCaculate/Lock ==
  FaultCnt : Inport
  Action Port : ActionPort  InitializeStates=reset  ActionPortLabel=elseif(u3 > 0)
  Constant : Constant  Value=20  OutDataTypeStr=uint16
  Constant1 : Constant  Value=2/TaskTimeBase.SpeedCtrl  OutDataTypeStr=uint16
  Constant2 : Constant  Value=65535  OutDataTypeStr=uint16
  Relational Operator : RelationalOperator  Operator=<  OutDataTypeStr=boolean  RndMeth=Simplest  InputSameDT=off
  Switch5 : Switch  Criteria=u2 > Threshold  SaturateOnIntegerOverflow=off  InputSameDT=off
  Interval : Outport  VectorParamsAs1DForOutWhenUnconnected=off
  wires:
  Constant/1 -> Relational Operator/2
  Relational Operator/1 -> Switch5/2
  Constant2/1 -> Switch5/3
  Constant1/1 -> Switch5/1
  FaultCnt/1 -> Relational Operator/1
  Switch5/1 -> Interval/1  "FaultType"

== system AppMain/MotorRestartAndFaultCnt/MotorFalutHandle/Subsystem/If Action Subsystem/RestartIntervalCaculate/Open ==
  FaultCnt : Inport
  Action Port : ActionPort  InitializeStates=reset  ActionPortLabel=elseif(u2 > 0)
  Constant : Constant  Value=20  OutDataTypeStr=uint16
  Constant1 : Constant  Value=2/TaskTimeBase.SpeedCtrl  OutDataTypeStr=uint16
  Constant2 : Constant  Value=65535  OutDataTypeStr=uint16
  Relational Operator : RelationalOperator  Operator=<  OutDataTypeStr=boolean  RndMeth=Simplest  InputSameDT=off
  Switch5 : Switch  Criteria=u2 > Threshold  SaturateOnIntegerOverflow=off  InputSameDT=off
  Interval : Outport  VectorParamsAs1DForOutWhenUnconnected=off
  wires:
  Constant/1 -> Relational Operator/2
  Relational Operator/1 -> Switch5/2
  Constant2/1 -> Switch5/3
  Constant1/1 -> Switch5/1
  FaultCnt/1 -> Relational Operator/1
  Switch5/1 -> Interval/1  "FaultType"

== system AppMain/MotorRestartAndFaultCnt/MotorFalutHandle/Subsystem/If Action Subsystem/RestartIntervalCaculate/Short ==
  FaultCnt : Inport
  Action Port : ActionPort  InitializeStates=reset  ActionPortLabel=if(u1 > 0)
  Constant : Constant  Value=20  OutDataTypeStr=uint16
  Constant1 : Constant  Value=2/TaskTimeBase.SpeedCtrl  OutDataTypeStr=uint16
  Constant2 : Constant  Value=65535  OutDataTypeStr=uint16
  Relational Operator : RelationalOperator  Operator=<  OutDataTypeStr=boolean  RndMeth=Simplest  InputSameDT=off
  Switch5 : Switch  Criteria=u2 > Threshold  SaturateOnIntegerOverflow=off  InputSameDT=off
  Interval : Outport  VectorParamsAs1DForOutWhenUnconnected=off
  wires:
  Constant/1 -> Relational Operator/2
  Relational Operator/1 -> Switch5/2
  Constant2/1 -> Switch5/3
  Constant1/1 -> Switch5/1
  FaultCnt/1 -> Relational Operator/1
  Switch5/1 -> Interval/1  "FaultType"

== system AppMain/PwmInTargetSpeedEval/NormalState/PwmInSpeedCtrl/DutySpeedCtrl/SpeedAndOutDelayEval/MaxSpeedLimtedByVoltage ==
  Voltage : Inport  OutDataTypeStr=int16
  1-D Lookup Table : Lookup_n-D  NumberOfTableDimensions=1  BreakpointsForDimension1=int16([170 240 320])  Table=int16([256 256 256])  TableDataTypeStr=Inherit: Inherit from 'Table data'  ExtrapMethod=Clip  InternalRulePriority=Speed  RndMeth=Simplest
  Constant : Constant  Value=CtrlConst.SpeedCtrl.PwmIn.TargetSpeed.Max  OutDataTypeStr=int16
  Constant1 : Constant  Value=256  OutDataTypeStr=int16
  Divide : Product  Inputs=**/
  MaxSpeed : Outport  VectorParamsAs1DForOutWhenUnconnected=off
  wires:
  Voltage/1 -> 1-D Lookup Table/1
  Constant/1 -> Divide/1
  1-D Lookup Table/1 -> Divide/2
  Divide/1 -> MaxSpeed/1
  Constant1/1 -> Divide/3

== system AppMain/PwmInTargetSpeedEval/NormalState/PwmInSpeedCtrl/PwmInNotShort/DutyFilter/Enabled Subsystem ==
  Duty : Inport
  DutyLast : Inport  Port=2  OutDataTypeStr=uint16
  DutyBufIn : Inport  Port=3
  Enable : EnablePort
  DutyFilter : Subsystem
      settings: RTWFcnNameOpts=Use subsystem name
  FilteredDuty : Outport  VectorParamsAs1DForOutWhenUnconnected=off
  Valid : Outport  Port=2  VectorParamsAs1DForOutWhenUnconnected=off
  DutyBufOut : Outport  Port=3  VectorParamsAs1DForOutWhenUnconnected=off
  wires:
  DutyFilter/3(Valid) -> Valid/1
  DutyFilter/1(FilteredDuty) -> FilteredDuty/1  "FilteredDuty"
  DutyLast/1 -> DutyFilter/2(FilteredDutyLast)  "DutyLast"
  Duty/1 -> DutyFilter/1(Duty)  "Duty"
  DutyBufIn/1 -> DutyFilter/3(DutyBufIn)  "Duty"
  DutyFilter/2(DutyBufOut) -> DutyBufOut/1

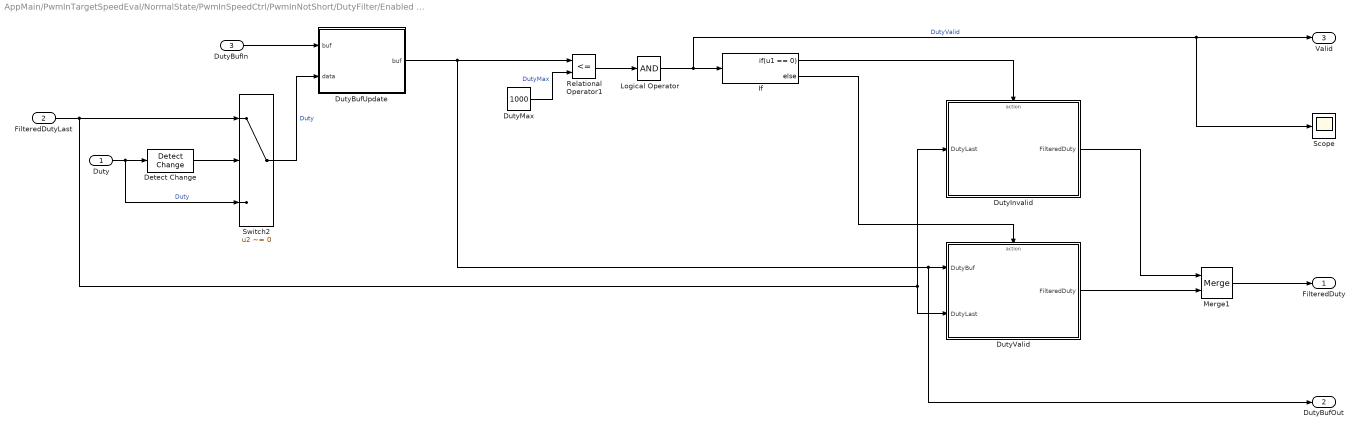
== system AppMain/PwmInTargetSpeedEval/NormalState/PwmInSpeedCtrl/PwmInNotShort/DutyFilter/Enabled Subsystem/DutyFilter ==
  Duty : Inport  OutDataTypeStr=uint16
  FilteredDutyLast : Inport  Port=2  OutDataTypeStr=uint16
  DutyBufIn : Inport  Port=3  OutDataTypeStr=uint16
  Detect Change : simulink/Logic and Bit Operations/Detect Change  vinit=0  OutDataTypeStr=boolean
  DutyBufUpdate : MATLAB Function  TreatAsAtomicUnit=on
      settings: RTWFcnNameOpts=Use subsystem name
  DutyInvalid : Subsystem  TreatAsAtomicUnit=on
  DutyMax : Constant  Value=1000  OutDataTypeStr=uint16
  DutyValid : Subsystem  TreatAsAtomicUnit=on
  If : If  IfExpression=u1 == 0
  Logical Operator : Logic  Inputs=1  AllPortsSameDT=off  OutDataTypeStr=boolean
  Merge1 : Merge
  Relational Operator1 : RelationalOperator  Operator=<=  OutDataTypeStr=boolean  RndMeth=Simplest  InputSameDT=off
  Scope : Scope
  Switch2 : Switch  Criteria=u2 ~= 0  SaturateOnIntegerOverflow=off  InputSameDT=off
  FilteredDuty : Outport  OutDataTypeStr=uint16  VectorParamsAs1DForOutWhenUnconnected=off
  DutyBufOut : Outport  Port=2  VectorParamsAs1DForOutWhenUnconnected=off
  Valid : Outport  Port=3  OutDataTypeStr=boolean  VectorParamsAs1DForOutWhenUnconnected=off
  wires:
  DutyBufUpdate/1(buf) -> DutyBufOut/1, DutyValid/1(DutyBuf), Relational Operator1/1
  Duty/1 -> Switch2/3, Detect Change/1  "Duty"
  DutyBufIn/1 -> DutyBufUpdate/1("buf ")
  DutyMax/1 -> Relational Operator1/2  "DutyMax"
  Relational Operator1/1 -> Logical Operator/1
  Logical Operator/1 -> If/1, Valid/1, Scope/1  "DutyValid"
  If/2 -> DutyValid/Action
  FilteredDutyLast/1 -> Switch2/1, DutyValid/2(DutyLast), DutyInvalid/1(DutyLast)
  DutyValid/1(FilteredDuty) -> Merge1/2
  Merge1/1 -> FilteredDuty/1
  DutyInvalid/1(FilteredDuty) -> Merge1/1
  If/1 -> DutyInvalid/Action
  Detect Change/1 -> Switch2/2
  Switch2/1 -> DutyBufUpdate/2(data)  "Duty"

== system AppMain/PwmInTargetSpeedEval/NormalState/PwmInSpeedCtrl/PwmInNotShort/DutyFilter/Enabled Subsystem/DutyFilter/DutyInvalid ==
  DutyLast : Inport  OutDataTypeStr=uint16
  Action Port : ActionPort  ActionPortLabel=if(u1 == 0)
  FilteredDuty : Outport  OutDataTypeStr=uint16  VectorParamsAs1DForOutWhenUnconnected=off
  wires:
  DutyLast/1 -> FilteredDuty/1

== system AppMain/PwmInTargetSpeedEval/NormalState/PwmInSpeedCtrl/PwmInNotShort/DutyFilter/Enabled Subsystem/DutyFilter/DutyValid ==
  DutyBuf : Inport  OutDataTypeStr=uint16
  DutyLast : Inport  Port=2  OutDataTypeStr=uint16
  Action Port : ActionPort  ActionPortLabel=else
  BufDataSameFirstCnt : MATLAB Function  TreatAsAtomicUnit=on
      settings: RTWFcnNameOpts=Use subsystem name
  DutySameCntTHR : Constant  Value=CtrlConst.SpeedCtrl.PwmIn.Duty.Filter.DutySameCntTHR  OutDataTypeStr=uint16  SampleTime=-1
  DutyTolerance : Constant  Value=CtrlConst.SpeedCtrl.PwmIn.Duty.Filter.DutyTolerance  OutDataTypeStr=uint16  SampleTime=-1
  Relational Operator : RelationalOperator  OutDataTypeStr=boolean  RndMeth=Simplest  InputSameDT=off
  Scope : Scope  NumInputPorts=3
  Selector : Selector  IndexMode=Zero-based  InputPortWidth=6  IndexOptions=Index vector (dialog)  Indices=0  OutputSizes=1
  Switch : Switch  Criteria=u2 > Threshold  SaturateOnIntegerOverflow=off  InputSameDT=off
  FilteredDuty : Outport  OutDataTypeStr=uint16  VectorParamsAs1DForOutWhenUnconnected=off
  wires:
  DutyLast/1 -> Switch/3
  Switch/1 -> FilteredDuty/1, Scope/2  "FilteredDuty"
  BufDataSameFirstCnt/1(samecnt) -> Relational Operator/1, Scope/1  "SameCnt"
  Selector/1 -> Switch/1, Scope/3  "Duty0"
  Relational Operator/1 -> Switch/2
  DutySameCntTHR/1 -> Relational Operator/2
  DutyBuf/1 -> BufDataSameFirstCnt/1(buf), Selector/1
  DutyTolerance/1 -> BufDataSameFirstCnt/2(tolerance)

== stateflow chart AppMain/MotorRestartAndFaultCnt/MotorFalutHandle/MotorFaultRecoverTimer/MotorRestartFSM ==
  state TimeCnt
    entry:
    TimeCnt = 1;
    RecoverEn = false;
    du:
    TimeCnt = TimeCnt + 1;
  state ReStart
    en:
    RecoverEn = true;
  (default) -> TimeCnt
  ReStart -> TimeCnt : [MotorRestartCompleted == true]
  TimeCnt -> ReStart : [TimeCnt >= TimeTHR && TimeTHR ~= 65535]
  data: TimeTHR input uint16; MotorRestartCompleted input boolean; TimeCnt local uint16 =uint16(0); RecoverEn output boolean =false

== stateflow chart AppMain/SleepMode/SleepMode ==
  state SleepWait
    SleepWait -> (junction 16)
    (junction 16) -> (junction 18) [order 1] : [SleepWaitTime < SleepWaitTimeTHR]
        | {SleepWaitTime = SleepWaitTime + 1;}
    (junction 16) -> (junction 22) [order 2]
    (junction 22) -> (junction 21) [order 1] : [SleepValid == true]
        | {ChipSleep = true;}
    (junction 22) -> (junction 24) [order 2] : {ChipReset = true;}
  state SleepValidFilter
    en:
    GoToSleep = false;
    ChipSleep = false;
    ChipReset = false;
    exit:
    GoToSleep = true;
    (junction 9) -> (junction 11) [order 1] : [SleepValid == true]
        | {SleepValidCnt = SleepValidCnt + 1;}
    SleepValidFilter -> (junction 9) [order 1]
    (junction 9) -> (junction 11) [order 2] : {SleepValidCnt =uint16( 0);}
  (default) -> SleepValidFilter
  SleepValidFilter -> SleepWait [order 1] : [SleepValid == true && SleepValidCnt >= SleepValidCntTHR]
      | {SleepWaitTime = uint16(1);}
  data: SleepValid input boolean; SleepWaitTime local uint16; GoToSleep output boolean; SleepValidCnt local uint16 =uint16(0); ChipSleep output boolean =false; ChipReset output boolean =false; SleepValidCntTHR input uint16; SleepWaitTimeTHR input uint16

== stateflow chart AppMain/FeedBack/StateKeep ==
  state TrueState
    en:
    State = true;
    FalseTime = 0;
    du:
    State = true;
    TrueState -> (junction 20) [order 1]
    (junction 20) -> (junction 22) [order 1] : [TrueTime > 0]
        | {TrueTime = TrueTime -1;}
    (junction 20) -> (junction 30) [order 2]
    (junction 32) -> (junction 22)
    (junction 30) -> (junction 32)
  state FalseState
    en:
    State = false;
    TrueTime=TrueKeepTime;
    FalseTime=FalseKeepTime;
    du:
    State = false;
    FalseState -> (junction 25) [order 1]
    (junction 25) -> (junction 27) [order 1] : [FalseTime > 0]
        | {FalseTime = FalseTime - 1;}
    (junction 25) -> (junction 35) [order 2]
    (junction 37) -> (junction 27)
    (junction 35) -> (junction 37) [order 1] : [TrueTime == 0]
        | {TrueTime=TrueKeepTime;
        | FalseTime=FalseKeepTime;}
    (junction 35) -> (junction 45) [order 2]
    (junction 47) -> (junction 37)
    (junction 45) -> (junction 47)
  (default) -> (junction 40) : {TrueTime=TrueKeepTime;
      | FalseTime=FalseKeepTime;}
  (junction 40) -> (junction 42) [order 2]
  (junction 40) -> FalseState [order 1] : [FalseTime ~= 0]
  (junction 42) -> TrueState
  TrueState -> FalseState [order 1] : [(TrueTime <= 1) &&  (FalseKeepTime > 0)]
  FalseState -> TrueState [order 1] : [FalseTime <= 1 && TrueTime > 0]
  data: State output boolean; BusSateCnt local uint16; FalseTime local uint16 =uint16(65535); TrueTime local uint16 =uint16(65535); FalseKeepTime input uint16; TrueKeepTime input uint16

== stateflow chart AppMain/FeedBack/FaultFeedBack/FeedBackTime ==
  state TimeJudge
    du:
    FeedBackNumberActual=FeedBackNumber;
    state FeedBackFiveBefore
      en:
      local_hightime=HighTime;
      local_lowtime=LowTime;
      FeedBackFlagLast=FeedBackFlag;
      FaultRecoverCnt=0;
      FeedBackNumberLast=FeedBackNumber;
      du:
      FeedBackFlagActual=FeedBackFlag;
      FeedBackNumberActual=FeedBackNumber;
      (junction 71) -> (junction 72) [order 1] : [FeedBackNumberActual~=FeedBackNumberLast]
          | {FaultRecoverCnt = FaultRecoverCnt + 1;}
      FeedBackFiveBefore -> (junction 71) [order 1]
      (junction 71) -> (junction 72) [order 2] : [FaultRecoverCnt>0]
          | {FaultRecoverCnt = FaultRecoverCnt - 1;}
      (junction 72) -> (junction 73) [order 1] : [FaultRecoverCnt > 50]
          | {FaultRecoverCnt=50}
      (junction 74) -> (junction 107) [order 1] : [FeedBackClearComplete==1]
          | {FeedBackClearEn=false;}
      (junction 73) -> (junction 74) : {TrueKeepTime=local_hightime;
          | FalseKeepTime=local_lowtime;
          | FaultRecoverCntOut=FaultRecoverCnt;}
      (junction 72) -> (junction 73) [order 2]
      (junction 71) -> (junction 72) [order 3] : {FaultRecoverCnt=0;}
      (junction 74) -> (junction 107) [order 2]
    state NewFaultJudge
      du:
      FeedBackClearEn=true;
    state FeedBackFiveAfter
      du:
      local_hightime=HighTime;
      local_lowtime=LowTime;
      FeedBackFlagLast=FeedBackFlag;
      FeedBackNumberActual=FeedBackNumber;
      FeedBackFiveAfter -> (junction 64) [order 1]
      (junction 64) -> (junction 65) : {TrueKeepTime=local_hightime;
          | FalseKeepTime=local_lowtime;}
    FeedBackFiveBefore -> NewFaultJudge [order 1] : [((FeedBackNumberActual~=FeedBackNumberLast)...
        | &&(FeedBackFlag==true))...
        | &&(FeedBackCnt>=5)...
        | &&(FaultRecoverCnt>=50)]
    (junction 62) -> FeedBackFiveBefore [order 1] : [(FeedBackCnt<5)...
        | &&(FeedBackFlag==true)]
    NewFaultJudge -> FeedBackFiveBefore : [FeedBackClearEn==true]
    (default) -> (junction 62)
    (junction 62) -> FeedBackFiveAfter [order 2]
    FeedBackFiveBefore -> FeedBackFiveAfter [order 2] : [(FeedBackCnt>=5)...
        | &&(FaultRecoverCnt>=50)]
    FeedBackFiveAfter -> FeedBackFiveBefore [order 1] : [((FeedBackCnt<5)...
        | &&(FeedBackFlag==true))]
  (default) -> TimeJudge
  data: HighTime input; LowTime input; local_hightime local; local_lowtime local; FalseKeepTime output; TrueKeepTime output; FaultRecoverCnt local uint16; FaultRecoverCntOut output; FeedBackCnt input uint16; FeedBackFlag input boolean; FeedBackFlagLast output; FeedBackClearComplete input; FeedBackClearEn output boolean; FeedBackNumber input; FeedBackNumberActual local; FeedBackNumberLast local; FeedBackFlagActual local

== matlab function AppMain/PwmInTargetSpeedEval/NormalState/PwmInSpeedCtrl/DutySpeedCtrl/SpeedAndOutDelayEval/SpeedCurve ==
  data: MaxSpeed input; MinSpeed input; Duty input; SectorLast input; Speed output; Delay output; Reset output; SectorNew output
function [Speed,Delay,Reset,SectorNew] = BufDataFirst2End(MaxSpeed, MinSpeed, Duty, SectorLast)
% # eml
if Duty >= 940
    Speed = int16(MaxSpeed);
elseif Duty >= 180
    Speed = int16((uint32(Duty) - uint32(180)) ...
    *(uint32(MaxSpeed) - uint32(MinSpeed)) ...
    /(uint32(940) - uint32(180)) ...
    +uint32(MinSpeed));
elseif Duty >=130
    Speed = int16(MinSpeed); 
elseif Duty >=80
    Speed = int16(0); 
else 
   Speed = int16(MaxSpeed);
end
    
        
Delay = uint16(0);
Reset = true;
SectorNew = uint16(SectorLast);

== matlab function AppMain/PwmInTargetSpeedEval/NormalState/PwmInSpeedCtrl/PwmInNotShort/DutyFilter/Enabled Subsystem/DutyFilter/DutyBufUpdate ==
  data: buf input; data input; buf output
function buf = BufDataFirst2End(buf,data)
% # eml
len = length(buf);
for i = 0 : len -2
    buf(len - i) = buf(len - i - 1);
end

buf(1) = data;

== matlab function AppMain/PwmInTargetSpeedEval/NormalState/PwmInSpeedCtrl/PwmInNotShort/DutyFilter/Enabled Subsystem/DutyFilter/DutyValid/BufDataSameFirstCnt ==
  data: buf input; samecnt output; tolerance input
function samecnt = BufDataSameFirstCnt(buf,tolerance)
if buf(1,1) >= tolerance
    min = buf(1,1) - tolerance;
else
    min = uint16(0);
end

max = buf(1,1) + tolerance;
if max > 1000
   max = uint16(1000); 
end

samecnt = uint16(1);
for i = 2:length(buf)
    if buf(i) >= min && buf(i) <= max
       samecnt = samecnt + 1; 
    end
end

== stateflow chart AppMain/PwmInTargetSpeedEval/NormalState/PwmInSpeedCtrl/PwmInNotShort/FreqValidJudge/FreqValidJudge ==
  state Invalid
    entry:
    Valid = false;
    ValidCnt = 1;
    Invalid -> (junction 37) [order 1] : {Valid = false;}
    (junction 37) -> (junction 38) [order 1] : [    (Freq <= FreqMax) ...
        | &&(Freq >= FreqMin)]
        | {ValidCnt = ValidCnt + 1;}
    (junction 37) -> (junction 38) [order 2] : {ValidCnt = 1;}
  state Valid
    entry:
    Valid = true;
    InvalidCnt = 1;
    Valid -> (junction 9) [order 1] : {Valid = true;}
    (junction 9) -> (junction 11) [order 1] : [ (Freq > FreqMax + FreqTolerance) ...
        | ||(Freq + FreqTolerance < FreqMin)]
        | {InvalidCnt = InvalidCnt + 1;}
    (junction 9) -> (junction 11) [order 2] : {InvalidCnt = 1; }
  (junction 56) -> Invalid
  (junction 54) -> (junction 56) [order 2]
  Valid -> Invalid [order 1] : [InvalidCnt >=FreqValidJudgeFilterTime]
  Invalid -> Valid [order 1] : [ValidCnt >=FreqValidJudgeFilterTime]
  (default) -> (junction 54)
  (junction 54) -> Valid [order 1] : [(Freq <= FreqMax + FreqTolerance) ...
      | &&(Freq + FreqTolerance >= FreqMin)]
  data: Freq input uint16; Valid output boolean =false; ValidLast local boolean =true; ValidCnt local uint16 =uint16(0); InvalidCnt local uint16 =uint16(0); InvalidLast local boolean =false; Invalid local boolean =false; FreqMin input uint16; FreqMax input uint16; FreqTolerance input uint16; FreqValidJudgeFilterTime input uint16

== stateflow chart AppMain/PwmInTargetSpeedEval/NormalState/PwmInSpeedCtrl/SpeedDelayOut/DelayOut ==
  state Delay
    Delay -> (junction 29) [order 1]
    (junction 29) -> (junction 30) [order 1] : [DelayCnt < DelayTHR]
        | {DelayCnt = DelayCnt + 1;
        | Out = OutLast;}
    (junction 29) -> (junction 31) [order 2]
    (junction 32) -> (junction 30)
    (junction 31) -> (junction 32) : {Out = In;}
  state Reset
    en:
    DelayCnt = 2;
    Out = OutLast;
  (default) -> Reset
  Reset -> Delay : [Rst == false]
  Delay -> Reset [order 1] : [Rst == true]
  data: DelayCnt local uint16 =uint16(0); In input int16; Out output int16 =int16(0); DelayTHR input uint16; Rst input boolean; OutLast input int16
